simulink model "Week3_problem2"  (R2020b)
settings: Solver=VariableStepAuto  StartTime=0.0  StopTime=10.0  RelTol=1e-3
settings Model: Creator=omkar  LastModifiedBy=omkar

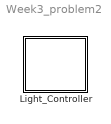
== system Week3_problem2 ==
  Light_Controller : Stateflow chart  TreatAsAtomicUnit=on

== stateflow chart Week3_problem2/Light_Controller ==
  state Stop
    y1=RED;
    y2=GREEN
  state StopForTraffic
    y1=RED;
    y2=GREEN;
  state StopToGo
    y1=RED;
    y2=YELLOW;
  state GoToStop
    y1=YELLOW;
    y2=RED;
  state Go
    y1=GREEN;
    y2=RED;
  (default) -> Stop
  Stop -> StopForTraffic : after(20,tick)
  StopForTraffic -> StopToGo : [sens]
  GoToStop -> Stop : after(3,tick)
  StopToGo -> Go : after(3,tick)
  Go -> GoToStop : after(10,tick)
